simulink model "myocyteNM_V4dyn"  (R2024b)
settings: Solver=ode1  StartTime=0.0  StopTime=restEnd  FixedStep=stepsize  RelTol=1e-3  EnableMultiTasking=on
values from neighbouring files (symbols this model uses):
  nm = 10    [restitution_run.m]
undefined symbols (not defined in the file or in its folder): duration, initial, trim
libraries: Libs_unified x1
settings Model: SimulationMode=accelerator  PauseTimes=10  Creator=wai484  LastModifiedBy=ball907
settings SolverCC: AlgebraicLoopSolver=TrustRegion
settings DataIOCC: SaveFormat=Array  SignalLogging=off  DSMLogging=off  SaveTime=off  ReturnWorkspaceOutputs=off
settings OptimizationCC: LifeSpan=inf  SimCompilerOptimization=on
settings DebuggingCC: SolverPrmCheckMsg=warning  UnconnectedInputMsg=warning  UnconnectedOutputMsg=warning  UnconnectedLineMsg=warning  SFUnexpectedBacktrackingDiag=warning  SFNoUnconditionalDefaultTransitionDiag=warning  SFExecutionAtInitializationDiag=none  ArithmeticOperatorsInVariantConditions=warning
settings HardwareCC: ProdBitPerPointer=32  ProdBitPerSizeT=32  ProdBitPerPtrDiffT=32  ProdLargestAtomicFloat=None  ProdIntDivRoundTo=Undefined  ProdEndianess=Unspecified  ProdWordSize=32  ProdHWDeviceType=32-bit Generic
settings ModelReferenceCC: EnableRefExpFcnMdlSchedulingChecks=on  PropagateSignalLabelsOutOfModel=off
settings SFSimCC: SimUseLocalCustomCode=off  CustomCodeUndefinedFunction=UseInterfaceOnly
settings RTWCC: RTWUseLocalCustomCode=off  BuildConfiguration=Faster Runs  GPUComputeCapability=3.5
settings CodeAppCC: StateflowObjectComments=on
settings GRTTargetCC: TargetLangStandard=C89/C90 (ANSI)
settings ConfigComp: CovMetricSettings=dw  CovSaveCumulativeToWorkspaceVar=on  CovSaveSingleToWorkspaceVar=on  CovExternalEMLEnable=off  CovSFcnEnable=off

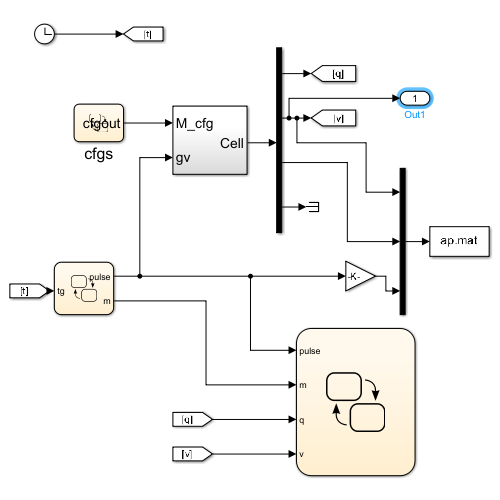
[thumbnail: Simulink's stored preview of the top-level diagram]
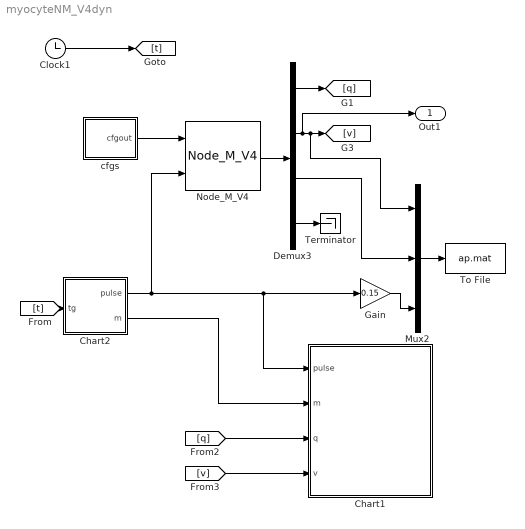
== system myocyteNM_V4dyn ==
  Chart1 : Stateflow chart  TreatAsAtomicUnit=on
  Chart2 : Stateflow chart  TreatAsAtomicUnit=on
  Clock1 : Clock
  Demux3 : Demux  Outputs=[1, 1, 1,2]
  Gain : Gain  Gain=0.15
  Mux2 : Mux  Inputs=3
  Node_M_V4 : Libs_unified/Node_M_V4  SystemSampleTime=-1  VariantActivationTime=update diagram  AllowFlexibleInterface=on  Latency=0  AutoFrameSizeCalculation=off
  Terminator : Terminator
  To File : ToFile  Filename=ap.mat  MatrixName=ap
  cfgs : Stateflow chart  TreatAsAtomicUnit=on
  Out1 : Outport
  wires:
  [q] -> Chart1/3(q)
  [v] -> Chart1/4(v)
  Chart2/1(pulse) -> Node_M_V4/2, Chart1/1(pulse), Gain/1
  Node_M_V4/1 -> Demux3/1
  Demux3/1 -> [q]
  Demux3/3 -> Mux2/2
  Demux3/2 -> Out1/1, Mux2/1, [v]
  Demux3/4 -> Terminator/1
  Mux2/1 -> To File/1
  Chart2/2(m) -> Chart1/2(m)
  Gain/1 -> Mux2/3
  Clock1/1 -> [t]
  [t] -> Chart2/1(tg)
  cfgs/1(cfgout) -> Node_M_V4/1

== stateflow chart myocyteNM_V4dyn/Chart2 ==
  state wait
  state pre1
    en:pulse=1000;
  state pace1
    en:m=m+1;
    pulse=1000;
  state pre0
    entry: pulse=0;
  state ready
  state pace0
    entry: pulse=0;
  state end
  (default) -> wait
  wait -> pre1 : [tg>=trim]{m=0;p=initial;}
  pre1 -> pre0 : after(duration,sec)
  ready -> pace1 : after(p-duration,sec)
  pre0 -> ready [order 1] : [p==t]
  pre0 -> pre1 [order 2] : after(p-duration,sec)/{p=p-trim;}
  pace0 -> pace1 [order 2] : after(p-duration,sec)
  pace1 -> pace0 : after(duration,sec)
  pace0 -> end [order 1] : [m>=nm]
  data: t parameter; nm parameter; pulse output; m output; tg input; p local; trim parameter; duration parameter; initial parameter

== stateflow chart myocyteNM_V4dyn/Chart1 ==
  state recording
    state APD0 [parallel]
      settings: executionOrder=1
      state end
      state wait
      state wait1st
      state q01
        du:
        t0=temporalCount (sec);
        ex:
        APD=t1+t0;
        ERP=t1;
      state activation
        du:
        t1=temporalCount (sec);
      (default) -> recording.APD0.wait
      recording.APD0.wait -> wait1st : [m==0 && q==0 && pulse>0]
      wait1st -> recording.APD0.activation : [q==3]/{vmax=v;}
      recording.APD0.activation -> recording.APD0.q01 : [q==0 ]
      recording.APD0.q01 -> recording.APD0.end : [q==0 &&v<=vmax*0.1]/{record(1,APD,ERP);}
    state APD10 [parallel]
      settings: executionOrder=3
      state wait
      state wait10th
      state end
      state ERP
      note: The 10th occurs in the ERP of 9th AP
      state waitpeak
      state q01
        du:
        t0=temporalCount (sec);
        ex:
        APD=t1+t0;
        ERP=t1;
      state activation
        du:
        t1=temporalCount (sec);
      (default) -> recording.APD10.wait
      recording.APD10.wait -> wait10th : [m==nm&&pulse>0 ]
      wait10th -> recording.APD10.ERP [order 1] : [pulse>0&&q==3]/{APD=0; ERP=0; record(nm,APD,ERP);}
      wait10th -> waitpeak [order 2] : [pulse>=0&&q<3]
      waitpeak -> recording.APD10.activation : [q==3]/{vmax=v;}
      recording.APD10.activation -> recording.APD10.q01 : [q==0 ]
      recording.APD10.q01 -> recording.APD10.end : [q==0 &&v<=vmax*0.1]/{record(nm,APD,ERP);}
    state DI [parallel]
      settings: executionOrder=2
      state savedi
        en:record1(DI);
      state pulseover
      state wait9
      state pulse
      note: The 10th occurs in the RRP of 8th or 9th AP
      note: The 9th occurs in the ERP of 8th AP
      state di
        du:
        DI=temporalCount (sec);
      state ERP
      state wait8
      pulse -> pulseover : [m==nm-1 && pulse==0&&q==3]/{vmax=v;}
      wait9 -> pulse [order 1] : [m==nm-1 && pulse>0 && q==0]
      pulseover -> savedi [order 1] : [m==nm&& pulse>0]{DI=0;}
      di -> savedi : [m==nm && pulse>0]
      wait8 -> wait9 : [m==nm-2 && q==3]/{vmax=v;}
      wait9 -> recording.DI.ERP [order 2] : [m==nm-1&& pulse>=0 && q==3]
      recording.DI.ERP -> pulseover
      pulseover -> di [order 2] : [m==nm-1 &&q==0 &&v<=vmax*0.1]
      (default) -> wait8
  (default) -> recording : /{DI=0;t0=0;t1=0; coder.extrinsic('assignin');}
  data: n function_input; apd function_input; erp function_input; di function_input; pulse input; m input; q input; v input; t0 local; vmax local; APD local; ERP local; DI local; t1 local; nm parameter
  function record (n,apd,erp):
    | function record (n,apd,erp)
    | 
    | coder.extrinsic('assignin')
    | if n==1
    |     assignin('base', 'APD0',apd);
    |     assignin('base', 'ERP0',erp);
    | else
    |     assignin('base', 'APD',apd);
    |     assignin('base', 'ERP',erp);
    |     
    | end
  function record1 (di):
    | function record1 (di)
    | 
    | coder.extrinsic('assignin')
    | 
    | assignin('base', 'DI',di);
    | 
    | 
    | end

== stateflow chart myocyteNM_V4dyn/cfgs ==
  settings: executeAtInitialization=1
  state Ini
  (default) -> Ini : {cfgout=auto;}
  data: cfg function_output; params parameter; cfgout output
  function cfg = auto:
    | function cfg = auto
    | 
    | BCL=params(1,1);
    | SD=params(1,2);
    | f1=params(1,3);
    | f2=params(1,4);
    | sigma1sq=params(1,5);
    | sigma2sq=params(1,6);
    | 
    | d2=params(1,7); 
    | erp_out=params(1,8);
    | d0=params(1,9); 
    | MDP=params(1,10);
    | VT_N=params(1,11); 
    | VR_N=params(1,12); 
    | Vh_out=params(1,13);
    | 
    | hr_out=params(1,14); 
    | hs_out=params(1,15);
    | s_out=params(1,16);
    | j_out=params(1,17);
    | m_out=params(1,18); 
    | 
    | h_out=params(1,19);
    | f_out=params(1,20);
    | 
    | r_out=params(1,21);
    | 
    | ax0=params(1,22);
    | ay0=params(1,23);
    | az0=params(1,24);
    |  
    | ax1=params(1,25);
    | ay1=params(1,26);
    | az1=params(1,27);
    |  
    | ax2=params(1,28);
    | ay2=params(1,29);
    | az2=params(1,30);
    |  
    | ax3=params(1,31);
    | ay3=params(1,32);
    | az3=params(1,33);
    |  
    | bx1=params(1,34);
    | by1=params(1,35);
    | bz1=params(1,36);
    | 
    | VR_M=params(1,37);
    | VT_M=params(1,38);
    | VO=params(1,39);
    |  
    | a=params(1,40);
    | b=params(1,41);
    | c=params(1,42);
    | d=params(1,43);
    | e=params(1,44);
    | x=params(1,45);
    | y=params(1,46);
    | 
    | Dij=params(1,47);
    | Dji=params(1,48);
    | 
    | 
    | cfg=[BCL, SD, f1,f2,sigma1sq, sigma2sq,d2,erp_out,d0,MDP,VT_N,VR_N,Vh_out,hr_out,hs_out,s_out,j_out,m_out,h_out,f_out,r_out,x,y,ax0,ay0,az0,ax1,ay1,az1,ax2,ay2,az2,ax3,ay3,az3,bx1,by1,bz1,VR_M,VT_M,VO,a,b,c,d,e,x,y,Dij,Dji];
    | end
